simulink model "FPGA_UART"  (R2024a)
settings: Solver=FixedStepDiscrete  StartTime=0.0  StopTime=0.05  RelTol=1e-3
values from neighbouring files (symbols this model uses):
  Ts = 1/Fs    (= 7.50007500075e-06)    [new_generation_coeff.m]    (also in simon_test.m; simple_fft_test.m = 1/F; testPSD_c2d.m; testPSD_simulink.m)
libraries: hdlsllib x78, simulink_extras x12, simulink x5
(part 2 of 2)

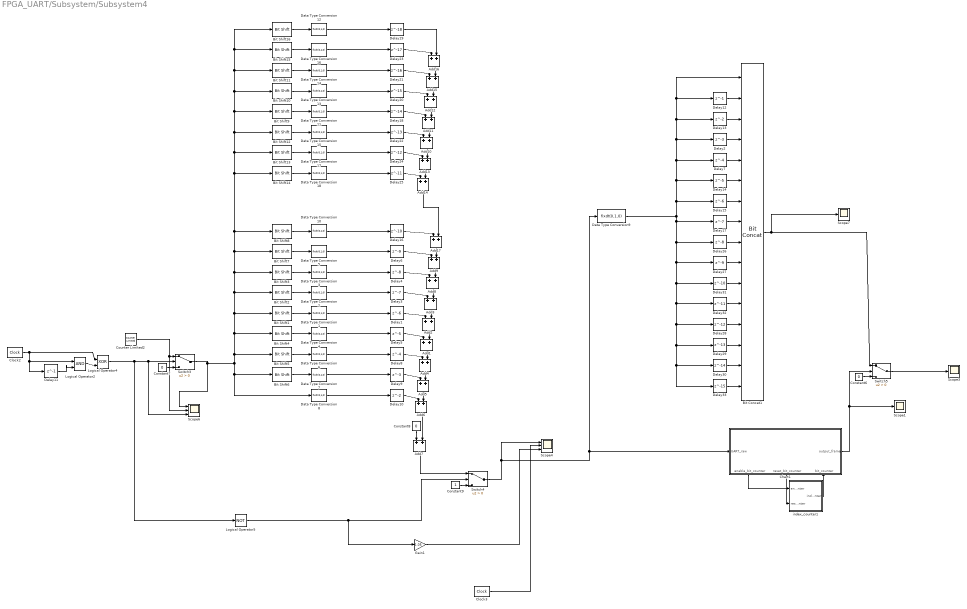
== system FPGA_UART/Subsystem/Subsystem4 ==
  Add{1..17} (17 alike) : Sum
  Bit Concat1 : hdlsllib/Logic and Bit Operations/Bit Concat  numInputs=16
  Bit Shift1 : hdlsllib/Logic and Bit Operations/Bit Shift  mode=Shift Right Logical  N=4
  Bit Shift10 : hdlsllib/Logic and Bit Operations/Bit Shift  mode=Shift Right Logical  N=13
  Bit Shift11 : hdlsllib/Logic and Bit Operations/Bit Shift  mode=Shift Right Logical  N=14
  Bit Shift12 : hdlsllib/Logic and Bit Operations/Bit Shift  mode=Shift Right Logical  N=11
  Bit Shift13 : hdlsllib/Logic and Bit Operations/Bit Shift  mode=Shift Right Logical  N=10
  Bit Shift14 : hdlsllib/Logic and Bit Operations/Bit Shift  mode=Shift Right Logical  N=9
  Bit Shift15 : hdlsllib/Logic and Bit Operations/Bit Shift  mode=Shift Right Logical  N=15
  Bit Shift16 : hdlsllib/Logic and Bit Operations/Bit Shift  mode=Shift Right Logical  N=16
  Bit Shift2 : hdlsllib/Logic and Bit Operations/Bit Shift  mode=Shift Right Logical  N=5
  Bit Shift3 : hdlsllib/Logic and Bit Operations/Bit Shift  mode=Shift Right Logical  N=6
  Bit Shift4 : hdlsllib/Logic and Bit Operations/Bit Shift  mode=Shift Right Logical  N=3
  Bit Shift5 : hdlsllib/Logic and Bit Operations/Bit Shift  mode=Shift Right Logical  N=2
  Bit Shift6 : hdlsllib/Logic and Bit Operations/Bit Shift  mode=Shift Right Logical  N=1
  Bit Shift7 : hdlsllib/Logic and Bit Operations/Bit Shift  mode=Shift Right Logical  N=7
  Bit Shift8 : hdlsllib/Logic and Bit Operations/Bit Shift  mode=Shift Right Logical  N=8
  Bit Shift9 : hdlsllib/Logic and Bit Operations/Bit Shift  mode=Shift Right Logical  N=12
  Chart1 : Stateflow chart  TreatAsAtomicUnit=on
      settings: PortSchema="{\"entries\":[{\"content\":{\"sides\":[{\"content\":{\"connectorIds\":[\"In2\"]},\"type\":\"ConnectorPlacement.EquallySpacedRectSide\",\"uuid\":\"2ee02e2e-a069-4e33-9774-57cdf73b0390\"},{\"content\":{\"connectorIds\":[\"Out1\"],\"side\":\"RIGHT\"},\"type\":\"ConnectorPlacement.EquallySpacedRectSide\",\"uuid\":\"21aeb1e6-6c65-4c00-a9b7-a995856e37fb\"},{\"content\":{\"side\":\"TOP\"},\"type\":\"ConnectorPlacement.EquallySpacedRectSide\",\"uuid\":\"d38f9540-57bf-4030-828c-0c58160bc96c\"},{\"content\":{\"connectorIds\":[\"Out2\",\"Out3\",\"In1\"],\"side\":\"BOTTOM\"},\"type\":\"ConnectorPlacement.EquallySpacedRectSide\",\"uuid\":\"4fe203c5-9b79-43fe-8008-8789174ca3d6\"}]},\"type\":\"ConnectorPlacement.EquallySpacedConnector\",\"uuid\":\"11cdfd4e-ecb7-4173-8729-c2a9bb2b5432\"}],\"packageUris\":[\"http://schema.mathworks.com/mf0/Connector/R2020b\"],\"version\":\"1.0\"}"
  Clock2 : simulink_extras/Flip Flops/Clock  period=Ts*18
  Clock3 : simulink_extras/Flip Flops/Clock  period=Ts
  Constant6 : Constant  Value=0  OutDataTypeStr=fixdt(0,4,0)  SampleTime=Ts
  Constant7 : Constant  Value=0  OutDataTypeStr=fixdt(0,4,0)  SampleTime=Ts
  Constant8 : Constant  Value=0  OutDataTypeStr=fixdt(0,4,0)  SampleTime=Ts
  Constant9 : Constant  OutDataTypeStr=fixdt(0,4,0)  SampleTime=Ts
  Counter Limited2 : simulink/Sources/Counter Limited  uplimit=65535  tsamp=Ts*18
  Data Type Conversion{1..8,10..18} (17 alike) : DataTypeConversion  OutDataTypeStr=fixdt(0,1,0)  SaturateOnIntegerOverflow=off  RndMeth=Floor
  Data Type Conversion9 : DataTypeConversion  OutDataTypeStr=fixdt(0,1,0)  RndMeth=Floor
  Delay1 : Delay  DelayLength=6  InitialCondition=0  SampleTime=Ts
  Delay10 : Delay  InitialCondition=0  SampleTime=Ts
  Delay11 : Delay  DelayLength=1  InitialCondition=0  SampleTime=Ts
  Delay12 : Delay  DelayLength=1  InitialCondition=0  SampleTime=Ts
  Delay13 : Delay  InitialCondition=0  SampleTime=Ts
  Delay14 : Delay  DelayLength=5  InitialCondition=0  SampleTime=Ts
  Delay15 : Delay  DelayLength=6  InitialCondition=0  SampleTime=Ts
  Delay16 : Delay  DelayLength=10  InitialCondition=0  SampleTime=Ts
  Delay17 : Delay  DelayLength=7  InitialCondition=0  SampleTime=Ts
  Delay18 : Delay  DelayLength=14  InitialCondition=0  SampleTime=Ts
  Delay19 : Delay  DelayLength=18  InitialCondition=0  SampleTime=Ts
  Delay2 : Delay  DelayLength=3  InitialCondition=0  SampleTime=Ts
  Delay20 : Delay  DelayLength=15  InitialCondition=0  SampleTime=Ts
  Delay21 : Delay  DelayLength=16  InitialCondition=0  SampleTime=Ts
  Delay22 : Delay  DelayLength=13  InitialCondition=0  SampleTime=Ts
  Delay23 : Delay  DelayLength=17  InitialCondition=0  SampleTime=Ts
  Delay24 : Delay  DelayLength=12  InitialCondition=0  SampleTime=Ts
  Delay25 : Delay  DelayLength=11  InitialCondition=0  SampleTime=Ts
  Delay26 : Delay  DelayLength=8  InitialCondition=0  SampleTime=Ts
  Delay27 : Delay  DelayLength=9  InitialCondition=0  SampleTime=Ts
  Delay28 : Delay  DelayLength=12  InitialCondition=0  SampleTime=Ts
  Delay29 : Delay  DelayLength=13  InitialCondition=0  SampleTime=Ts
  Delay3 : Delay  DelayLength=7  InitialCondition=0  SampleTime=Ts
  Delay30 : Delay  DelayLength=14  InitialCondition=0  SampleTime=Ts
  Delay31 : Delay  DelayLength=10  InitialCondition=0  SampleTime=Ts
  Delay32 : Delay  DelayLength=11  InitialCondition=0  SampleTime=Ts
  Delay33 : Delay  DelayLength=15  InitialCondition=0  SampleTime=Ts
  Delay4 : Delay  DelayLength=8  InitialCondition=0  SampleTime=Ts
  Delay5 : Delay  DelayLength=5  InitialCondition=0  SampleTime=Ts
  Delay6 : Delay  DelayLength=9  InitialCondition=0  SampleTime=Ts
  Delay7 : Delay  DelayLength=4  InitialCondition=0  SampleTime=Ts
  Delay8 : Delay  DelayLength=4  InitialCondition=0  SampleTime=Ts
  Delay9 : Delay  DelayLength=3  InitialCondition=0  SampleTime=Ts
  Gain1 : Gain  Gain=1.05
  Logical Operator2 : Logic  IconShape=distinctive  AllPortsSameDT=off  OutDataTypeStr=boolean
  Logical Operator4 : Logic  Operator=XOR  IconShape=distinctive  AllPortsSameDT=off  OutDataTypeStr=boolean
  Logical Operator5 : Logic  Operator=NOT  IconShape=distinctive  AllPortsSameDT=off  OutDataTypeStr=boolean
  Scope1 : Scope
  Scope3 : Scope
  Scope4 : Scope  NumInputPorts=3
  Scope6 : Scope  NumInputPorts=3
  Scope7 : Scope
  Switch3 : Switch  Criteria=u2 > Threshold  SaturateOnIntegerOverflow=off  InputSameDT=off
  Switch4 : Switch  Criteria=u2 > Threshold  SaturateOnIntegerOverflow=off  InputSameDT=off
  Switch5 : Switch  Criteria=u2 > Threshold  SaturateOnIntegerOverflow=off  InputSameDT=off  OutDataTypeStr=Inherit: Same as first input
  index_counter1 : Subsystem
  wires:
  Delay26/1 -> Bit Concat1/9
  Delay27/1 -> Bit Concat1/10
  Delay31/1 -> Bit Concat1/11
  Delay32/1 -> Bit Concat1/12
  Delay28/1 -> Bit Concat1/13
  Delay29/1 -> Bit Concat1/14
  Delay30/1 -> Bit Concat1/15
  Delay33/1 -> Bit Concat1/16
  Delay17/1 -> Bit Concat1/8
  Delay15/1 -> Bit Concat1/7
  Delay14/1 -> Bit Concat1/6
  Delay7/1 -> Bit Concat1/5
  Delay2/1 -> Bit Concat1/4
  Delay13/1 -> Bit Concat1/3
  Delay12/1 -> Bit Concat1/2
  Add14/1 -> Add17/2
  Add17/1 -> Add9/2
  Delay16/1 -> Add17/1
  Add13/1 -> Add14/2
  Delay24/1 -> Add13/1
  Delay22/1 -> Add10/1
  Bit Shift12/1 -> Data Type Conversion15/1
  Bit Shift14/1 -> Data Type Conversion18/1
  Delay25/1 -> Add14/1
  Data Type Conversion17/1 -> Delay24/1
  Bit Shift13/1 -> Data Type Conversion17/1
  Data Type Conversion18/1 -> Delay25/1
  Data Type Conversion15/1 -> Delay22/1
  Data Type Conversion11/1 -> Delay18/1
  Bit Shift9/1 -> Data Type Conversion11/1
  Add10/1 -> Add13/2
  Delay20/1 -> Add12/1
  Bit Shift10/1 -> Data Type Conversion13/1
  Data Type Conversion13/1 -> Delay20/1
  Data Type Conversion14/1 -> Delay21/1
  Bit Shift11/1 -> Data Type Conversion14/1
  Delay21/1 -> Add15/1
  Delay23/1 -> Add16/1
  Bit Shift15/1 -> Data Type Conversion16/1
  Data Type Conversion16/1 -> Delay23/1
  Add11/1 -> Add10/2
  Delay18/1 -> Add11/1
  Add12/1 -> Add11/2
  Add15/1 -> Add12/2
  Data Type Conversion12/1 -> Delay19/1
  Switch3/1 -> Scope6/1, Bit Shift6/1, Data Type Conversion8/1, Bit Shift5/1, Bit Shift4/1, Bit Shift1/1, Bit Shift2/1, Bit Shift3/1, Bit Shift7/1, Bit Shift8/1, Bit Shift14/1, Bit Shift13/1, Bit Shift12/1, Bit Shift9/1, Bit Shift10/1, Bit Shift11/1, Bit Shift16/1, Bit Shift15/1
  Bit Shift16/1 -> Data Type Conversion12/1
  Add16/1 -> Add15/2
  Delay19/1 -> Add16/2
  Data Type Conversion9/1 -> Delay15/1, Delay14/1, Delay7/1, Delay2/1, Delay13/1, Bit Concat1/1, Delay12/1, Delay17/1, Delay26/1, Delay27/1, Delay31/1, Delay32/1, Delay28/1, Delay29/1, Delay30/1, Delay33/1
  Add9/1 -> Add8/2
  Bit Shift8/1 -> Data Type Conversion10/1
  Data Type Conversion10/1 -> Delay16/1
  Add8/1 -> Add3/2
  Add3/1 -> Add2/2
  Delay1/1 -> Add2/1
  Add2/1 -> Add1/2
  Data Type Conversion5/1 -> Delay6/1
  Bit Shift7/1 -> Data Type Conversion5/1
  Delay6/1 -> Add9/1
  Delay4/1 -> Add8/1
  Bit Shift3/1 -> Data Type Conversion3/1
  Data Type Conversion3/1 -> Delay4/1
  Data Type Conversion2/1 -> Delay3/1
  Bit Shift2/1 -> Data Type Conversion2/1
  Delay3/1 -> Add3/1
  Add1/1 -> Add4/2
  Bit Shift1/1 -> Data Type Conversion1/1
  Data Type Conversion1/1 -> Delay1/1
  Data Type Conversion4/1 -> Delay5/1
  Add6/1 -> Add7/2
  Data Type Conversion7/1 -> Delay9/1
  Bit Shift5/1 -> Data Type Conversion6/1
  Delay11/1 -> Logical Operator2/2
  Chart1/3(reset_bit_counter) -> index_counter1/2(reset_bit_counter)
  Constant9/1 -> Switch4/3
  Logical Operator2/1 -> Logical Operator4/2
  Constant7/1 -> Switch3/3
  Delay10/1 -> Add6/1
  Data Type Conversion6/1 -> Delay8/1
  Add5/1 -> Add6/2
  Gain1/1 -> Scope4/3
  Switch5/1 -> Scope3/1
  Data Type Conversion8/1 -> Delay10/1
  Delay9/1 -> Add5/1
  Bit Shift6/1 -> Data Type Conversion7/1
  Clock3/1 -> Scope4/2
  Bit Shift4/1 -> Data Type Conversion4/1
  Counter Limited2/1 -> Switch3/1, Scope6/2
  Add7/1 -> Switch4/1
  Logical Operator5/1 -> Switch4/2, Gain1/1
  Delay5/1 -> Add1/1
  Logical Operator4/1 -> Switch3/2, Scope6/3, Logical Operator5/1
  Delay8/1 -> Add4/1
  index_counter1/1(index_counter) -> Chart1/1(bit_counter)
  Chart1/2(enable_bit_counter) -> index_counter1/1(enable_bit_counter)
  Switch4/1 -> Scope4/1, Data Type Conversion9/1, Chart1/2(UART_raw)
  Chart1/1(output_frame) -> Switch5/2, Scope1/1
  Constant8/1 -> Add7/1
  Clock2/1 -> Logical Operator4/1, Logical Operator2/1, Delay11/1
  Add4/1 -> Add5/2
  Bit Concat1/1 -> Switch5/1, Scope7/1
  Constant6/1 -> Switch5/3

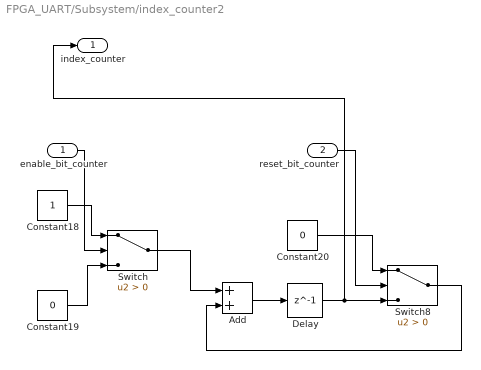
== system FPGA_UART/Subsystem/index_counter2 ==
  enable_bit_counter : Inport
  reset_bit_counter : Inport  Port=2
  Add : Sum  OutDataTypeStr=Inherit: Same as first input
  Constant18 : Constant  OutDataTypeStr=fixdt(0,8,0)  SampleTime=Ts
  Constant19 : Constant  Value=0  OutDataTypeStr=fixdt(0,8,0)  SampleTime=Ts
  Constant20 : Constant  Value=0  OutDataTypeStr=fixdt(0,8,0)  SampleTime=Ts
  Delay : Delay  DelayLength=1  InitialCondition=0  SampleTime=Ts
  Switch : Switch  Criteria=u2 > Threshold  SaturateOnIntegerOverflow=off  InputSameDT=off  OutDataTypeStr=Inherit: Same as first input
  Switch8 : Switch  Criteria=u2 > Threshold  SaturateOnIntegerOverflow=off  InputSameDT=off  OutDataTypeStr=Inherit: Same as first input
  index_counter : Outport
  wires:
  Constant19/1 -> Switch/3
  Switch8/1 -> Add/2
  Switch/1 -> Add/1
  Delay/1 -> index_counter/1, Switch8/3
  reset_bit_counter/1 -> Switch8/2
  Add/1 -> Delay/1
  Constant20/1 -> Switch8/1
  Constant18/1 -> Switch/1
  enable_bit_counter/1 -> Switch/2

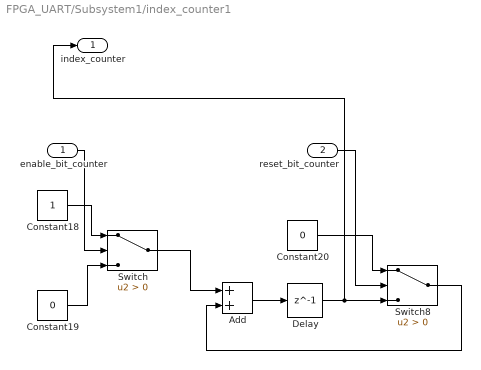
== system FPGA_UART/Subsystem1/index_counter1 ==
  enable_bit_counter : Inport
  reset_bit_counter : Inport  Port=2
  Add : Sum  OutDataTypeStr=fixdt(0,4,0)  AccumDataTypeStr=fixdt(0,4,0)
  Constant18 : Constant  OutDataTypeStr=fixdt(0,4,0)  SampleTime=Ts
  Constant19 : Constant  Value=0  OutDataTypeStr=fixdt(0,4,0)  SampleTime=Ts
  Constant20 : Constant  Value=0  OutDataTypeStr=fixdt(0,4,0)  SampleTime=Ts
  Delay : Delay  DelayLength=1  InitialCondition=0  SampleTime=Ts
  Switch : Switch  Criteria=u2 > Threshold  OutDataTypeStr=fixdt(0,4,0)  SaturateOnIntegerOverflow=off  InputSameDT=off
  Switch8 : Switch  Criteria=u2 > Threshold  OutDataTypeStr=fixdt(0,4,0)  SaturateOnIntegerOverflow=off  InputSameDT=off
  index_counter : Outport
  wires:
  enable_bit_counter/1 -> Switch/2
  Constant18/1 -> Switch/1
  Constant20/1 -> Switch8/1
  Add/1 -> Delay/1
  reset_bit_counter/1 -> Switch8/2
  Delay/1 -> Switch8/3, index_counter/1
  Switch/1 -> Add/1
  Switch8/1 -> Add/2
  Constant19/1 -> Switch/3

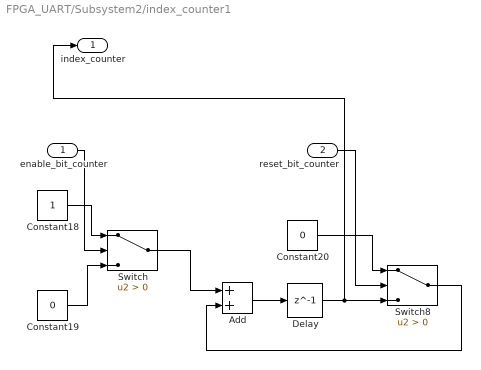
== system FPGA_UART/Subsystem2/index_counter1 ==
  enable_bit_counter : Inport
  reset_bit_counter : Inport  Port=2
  Add : Sum  OutDataTypeStr=Inherit: Same as first input
  Constant18 : Constant  OutDataTypeStr=fixdt(0,8,0)  SampleTime=Ts
  Constant19 : Constant  Value=0  OutDataTypeStr=fixdt(0,8,0)  SampleTime=Ts
  Constant20 : Constant  Value=0  OutDataTypeStr=fixdt(0,8,0)  SampleTime=Ts
  Delay : Delay  DelayLength=1  InitialCondition=0  SampleTime=Ts
  Switch : Switch  Criteria=u2 > Threshold  SaturateOnIntegerOverflow=off  InputSameDT=off  OutDataTypeStr=Inherit: Same as first input
  Switch8 : Switch  Criteria=u2 > Threshold  SaturateOnIntegerOverflow=off  InputSameDT=off  OutDataTypeStr=Inherit: Same as first input
  index_counter : Outport
  wires:
  enable_bit_counter/1 -> Switch/2
  Constant18/1 -> Switch/1
  Constant20/1 -> Switch8/1
  Add/1 -> Delay/1
  reset_bit_counter/1 -> Switch8/2
  Delay/1 -> Switch8/3, index_counter/1
  Switch/1 -> Add/1
  Switch8/1 -> Add/2
  Constant19/1 -> Switch/3

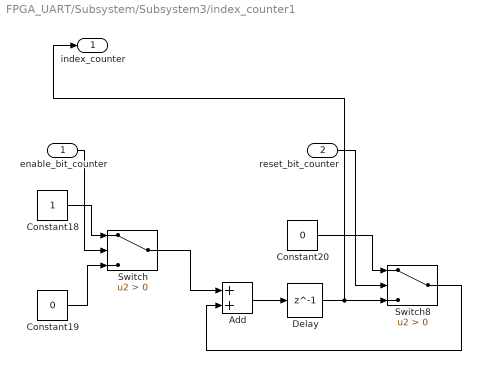
== system FPGA_UART/Subsystem/Subsystem3/index_counter1 ==
  enable_bit_counter : Inport
  reset_bit_counter : Inport  Port=2
  Add : Sum  OutDataTypeStr=fixdt(0,4,0)  AccumDataTypeStr=fixdt(0,4,0)
  Constant18 : Constant  OutDataTypeStr=fixdt(0,4,0)  SampleTime=Ts
  Constant19 : Constant  Value=0  OutDataTypeStr=fixdt(0,4,0)  SampleTime=Ts
  Constant20 : Constant  Value=0  OutDataTypeStr=fixdt(0,4,0)  SampleTime=Ts
  Delay : Delay  DelayLength=1  InitialCondition=0  SampleTime=Ts
  Switch : Switch  Criteria=u2 > Threshold  OutDataTypeStr=fixdt(0,4,0)  SaturateOnIntegerOverflow=off  InputSameDT=off
  Switch8 : Switch  Criteria=u2 > Threshold  OutDataTypeStr=fixdt(0,4,0)  SaturateOnIntegerOverflow=off  InputSameDT=off
  index_counter : Outport
  wires:
  enable_bit_counter/1 -> Switch/2
  Constant18/1 -> Switch/1
  Constant20/1 -> Switch8/1
  Add/1 -> Delay/1
  reset_bit_counter/1 -> Switch8/2
  Delay/1 -> Switch8/3, index_counter/1
  Switch/1 -> Add/1
  Switch8/1 -> Add/2
  Constant19/1 -> Switch/3

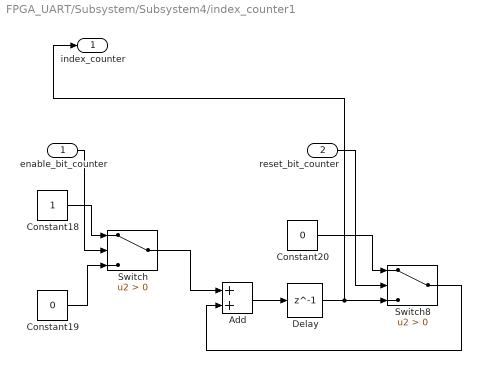
== system FPGA_UART/Subsystem/Subsystem4/index_counter1 ==
  enable_bit_counter : Inport
  reset_bit_counter : Inport  Port=2
  Add : Sum  OutDataTypeStr=Inherit: Same as first input
  Constant18 : Constant  OutDataTypeStr=fixdt(0,8,0)  SampleTime=Ts
  Constant19 : Constant  Value=0  OutDataTypeStr=fixdt(0,8,0)  SampleTime=Ts
  Constant20 : Constant  Value=0  OutDataTypeStr=fixdt(0,8,0)  SampleTime=Ts
  Delay : Delay  DelayLength=1  InitialCondition=0  SampleTime=Ts
  Switch : Switch  Criteria=u2 > Threshold  SaturateOnIntegerOverflow=off  InputSameDT=off  OutDataTypeStr=Inherit: Same as first input
  Switch8 : Switch  Criteria=u2 > Threshold  SaturateOnIntegerOverflow=off  InputSameDT=off  OutDataTypeStr=Inherit: Same as first input
  index_counter : Outport
  wires:
  enable_bit_counter/1 -> Switch/2
  Constant18/1 -> Switch/1
  Constant20/1 -> Switch8/1
  Add/1 -> Delay/1
  reset_bit_counter/1 -> Switch8/2
  Delay/1 -> Switch8/3, index_counter/1
  Switch/1 -> Add/1
  Switch8/1 -> Add/2
  Constant19/1 -> Switch/3

== stateflow chart FPGA_UART/Subsystem/Subsystem4/Chart1 ==
  state wait_on_bit
    entry:
    output_frame = false;
    enable_bit_counter = false;
    reset_bit_counter = true;
  state wait_for_bits_in_frame
    entry:
    output_frame = false;
    enable_bit_counter = true;
    reset_bit_counter = false;
  state send_frame_state
    entry:
    output_frame = true;
    enable_bit_counter = false;
    reset_bit_counter = true;
  (default) -> wait_on_bit
  wait_on_bit -> wait_for_bits_in_frame : [UART_raw == 0]
  (junction 11) -> wait_on_bit
  wait_for_bits_in_frame -> send_frame_state : [bit_counter == 16]
  send_frame_state -> (junction 11)
  data: output_frame output; bit_counter input; UART_raw input; enable_bit_counter output; reset_bit_counter output

== stateflow chart FPGA_UART/Chart1 ==
  state wait_on_bit
    entry:
    output_frame = false;
    enable_bit_counter = false;
    reset_bit_counter = true;
  state wait_for_bits_in_frame
    entry:
    output_frame = false;
    enable_bit_counter = true;
    reset_bit_counter = false;
  state send_frame_state
    entry:
    output_frame = true;
    enable_bit_counter = false;
    reset_bit_counter = true;
  (default) -> wait_on_bit
  wait_on_bit -> wait_for_bits_in_frame : [UART_raw == 0]
  (junction 11) -> wait_on_bit
  wait_for_bits_in_frame -> send_frame_state : [bit_counter == 16]
  send_frame_state -> (junction 11)
  data: output_frame output; bit_counter input; UART_raw input; enable_bit_counter output; reset_bit_counter output

== stateflow chart FPGA_UART/Subsystem1/Chart1 ==
  state wait_on_bit
    entry:
    output_frame = false;
    enable_bit_counter = false;
    reset_bit_counter = true;
  state wait_for_bits_in_frame
    entry:
    output_frame = false;
    enable_bit_counter = true;
    reset_bit_counter = false;
  state send_frame_state
    entry:
    output_frame = true;
    enable_bit_counter = false;
    reset_bit_counter = true;
  (default) -> wait_on_bit
  wait_on_bit -> wait_for_bits_in_frame : [UART_raw == 0]
  (junction 11) -> wait_on_bit
  wait_for_bits_in_frame -> send_frame_state : [bit_counter == 3]
  send_frame_state -> (junction 11)
  data: output_frame output; bit_counter input; UART_raw input; enable_bit_counter output; reset_bit_counter output

== stateflow chart FPGA_UART/Subsystem/Chart2 ==
  state wait_on_bit
    entry:
    output_frame = false;
    enable_bit_counter = false;
    reset_bit_counter = true;
  state wait_for_bits_in_frame
    entry:
    output_frame = false;
    enable_bit_counter = true;
    reset_bit_counter = false;
  state send_frame_state
    entry:
    output_frame = true;
    enable_bit_counter = false;
    reset_bit_counter = true;
  (default) -> wait_on_bit
  wait_on_bit -> wait_for_bits_in_frame : [UART_raw == 0]
  (junction 11) -> wait_on_bit
  wait_for_bits_in_frame -> send_frame_state : [bit_counter == 16]
  send_frame_state -> (junction 11)
  data: output_frame output; bit_counter input; UART_raw input; enable_bit_counter output; reset_bit_counter output

== stateflow chart FPGA_UART/Subsystem2/Chart1 ==
  state wait_on_bit
    entry:
    output_frame = false;
    enable_bit_counter = false;
    reset_bit_counter = true;
  state wait_for_bits_in_frame
    entry:
    output_frame = false;
    enable_bit_counter = true;
    reset_bit_counter = false;
  state send_frame_state
    entry:
    output_frame = true;
    enable_bit_counter = false;
    reset_bit_counter = true;
  (default) -> wait_on_bit
  wait_on_bit -> wait_for_bits_in_frame : [UART_raw == 0]
  (junction 11) -> wait_on_bit
  wait_for_bits_in_frame -> send_frame_state : [bit_counter == 16]
  send_frame_state -> (junction 11)
  data: output_frame output; bit_counter input; UART_raw input; enable_bit_counter output; reset_bit_counter output

== stateflow chart FPGA_UART/Subsystem/Subsystem3/Chart1 ==
  state wait_on_bit
    entry:
    output_frame = false;
    enable_bit_counter = false;
    reset_bit_counter = true;
  state wait_for_bits_in_frame
    entry:
    output_frame = false;
    enable_bit_counter = true;
    reset_bit_counter = false;
  state send_frame_state
    entry:
    output_frame = true;
    enable_bit_counter = false;
    reset_bit_counter = true;
  (default) -> wait_on_bit
  wait_on_bit -> wait_for_bits_in_frame : [UART_raw == 0]
  (junction 11) -> wait_on_bit
  wait_for_bits_in_frame -> send_frame_state : [bit_counter == 3]
  send_frame_state -> (junction 11)
  data: output_frame output; bit_counter input; UART_raw input; enable_bit_counter output; reset_bit_counter output
